simulink model "part1"  (R2024a)
settings: Solver=VariableStepAuto  StartTime=0.0  StopTime=10.0  RelTol=1e-3
values from neighbouring files (symbols this model uses):
  d1 = exp(-T/T1)    [calc.m]    (also in first_calc.m)
  d2 = exp(-T/T2)    [calc.m]    (also in first_calc.m)
  q0 = 18    [calc.m]    (also in first_calc.m = 2)
  T = T1/2    (= 0.225)    [calc.m]    (also in first_calc.m; second_calc.m = 0.2)
  T1 = 0.45    [calc.m]    (also in first_calc.m)
  T2 = 1.35    [calc.m]    (also in first_calc.m)
settings Model: Creator=ventus  LastModifiedBy=ventus

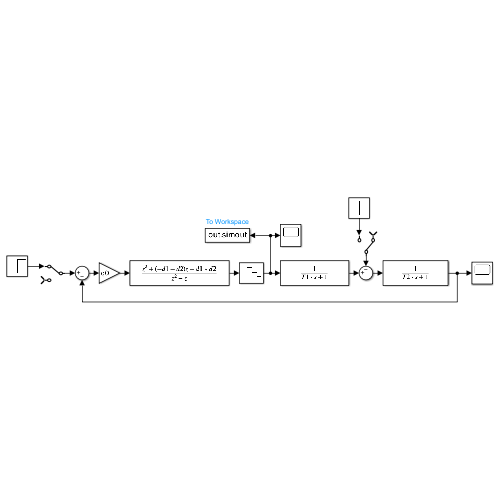
[thumbnail: Simulink's stored preview of the top-level diagram]
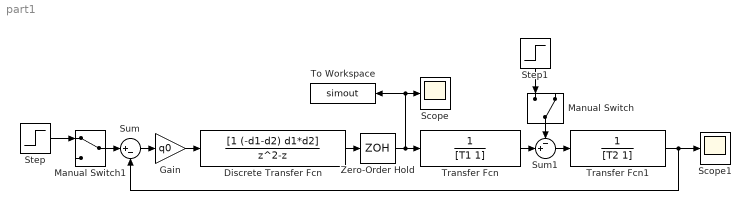
== system part1 ==
  Discrete Transfer Fcn : DiscreteTransferFcn  Numerator=[1 (-d1-d2) d1*d2]  Denominator=[1 -1 0]
  Gain : Gain  Gain=q0
  Manual Switch : ManualSwitch  CurrentSetting=0
  Manual Switch1 : ManualSwitch
  Scope : Scope
  Scope1 : Scope
  Step : Step  SampleTime=0
  Step1 : Step  SampleTime=0
  Sum : Sum  Inputs=|+-
  Sum1 : Sum  Inputs=-+|
  To Workspace : ToWorkspace  VariableName=simout  SaveFormat=Timeseries  SampleTime=-1
  Transfer Fcn : TransferFcn  Denominator=[T1 1]
  Transfer Fcn1 : TransferFcn  Denominator=[T2 1]
  Zero-Order Hold : ZeroOrderHold  SampleTime=T
  wires:
  Step/1 -> Manual Switch1/1
  Manual Switch1/1 -> Sum/1
  Sum/1 -> Gain/1
  Zero-Order Hold/1 -> To Workspace/1, Scope/1, Transfer Fcn/1
  Transfer Fcn/1 -> Sum1/2
  Manual Switch/1 -> Sum1/1
  Step1/1 -> Manual Switch/1
  Sum1/1 -> Transfer Fcn1/1
  Transfer Fcn1/1 -> Scope1/1, Sum/2
  Discrete Transfer Fcn/1 -> Zero-Order Hold/1
  Gain/1 -> Discrete Transfer Fcn/1
